simulink model "CML_Dyanmic_Sensory_Weighting"  (R2015a)
settings: Solver=ode4  SolverMode=MultiTasking  StartTime=0.0  StopTime=inf  FixedStep=BKIN_STEP_TIME  RelTol=1e-3
StartFcn:
  |  warndlg('Dexterit-E models cannot run under simulation. Please compile your model and run it from within Dexterit-E.');set_param(bdroot,'SimulationCommand','stop')
model workspace (MAT data in the model file):
  col_x = 1
  col_y = 2
  RADIUS_VIS = 3
  COLOR_INIT = 4
  START_TARGET_COL = 1
  DELAY_POST_TRIAL_COL = 17
  BKIN_STEP_TIME = 0.00025
  COLOR_MOVE = 5
  START_WAIT_TIME_COL = 2
  STIM_DUR_COL = 13
  MAX_MOVE_TIME_COL = 14
  HOLD_TIME_COL = 15
  E_START_TRIAL = 2
  E_START_REACHED = 4
  E_MOVED_EARLY = 21
  E_GO_CUE = 9
  E_MOVE_TIMEOUT = 23
  E_HOLDING_STILL = 12
  E_END_TRIAL = 14
  CONTROL_PT3_COL = 10
  STROKE_WIDTH = 6
  K_HAND_VEL = 1
  E_MOVE_ON = 10
  CUE_TYPE_COL = 6
  HAND_VIS_COL = 5
  K_HOLDTIME = 2
  K_ROBOT_RAMP_TIME = 3
  E_ROBOT_RETURN_TO_START = 33
  E_ENABLED_CONTROLLER = 31
  K_TIME_TO_START = 4
  E_RETURN_TO_START = 35
  E_HOLD_POS = 37
  E_INCREMENTING_TSTEP1 = 6
  E_INCREMENTING_TSTEP2 = 7
  E_INCREMENTING_TSTEP3 = 8
  CONTROL_PT0_COL = 7
  BKIN_KINEMATIC_FRAME_SIZE = 400
  E_NO_EVENT = 0
  E_BUTTON_ON = 40
  CONTROL_PTV1_COL = 8
  CONTROL_PTV2_COL = 9
  CONTROL_PTP1_COL = 11
  CONTROL_PTP2_COL = 12
  REACH_TARGET_COL = 3
  VIS_TARGET_COL = 4
  RADIUS_LOGICAL = 7
  FEEDBACK_TIME_COL = 16
  K_HAND_TARGET = 5
  E_SHOW_FEEDBACK = 16
  K_MIDPOINTY = 6
  K_MIDPOINT_Y = 6
  K_ARC_FDBK_TARGET = 7
  TEXT1 = 8
  TEXT2 = 9
  TEXT3 = 10
  K_CUE_TARGET = 8
  CONTINUE = 4
  TEXT4 = 11
  E_PAUSE = 41
libraries: slrtlib x10, Video x9, General x3, KINARM_general x3, KINARM_loads x2, xpcnilib x1
(part 2 of 2)

== matlab function CML_Dyanmic_Sensory_Weighting/BezierCurve/Bezier_fnc ==
  data: startxy input; segCount input; posV output; posP output; VCODE input; VCODE_mod output; t input; target_rows input; Ptarget_rows input; control_points input; col_xy input
function [posV,posP,VCODE_mod] = fcn(startxy,segCount,VCODE,t,target_rows,Ptarget_rows,control_points,col_xy)
%#codegen

%VCODE_mod = [VCODE; VCODE];
VCODE_mod = VCODE;


%startxy is the absolute starting point for the segment

%Vtarget_rows and Ptarget_rows share the same first target so we
%just have to ask about the remaining ones

%find all the nonzero (valid) control points
target_rows = target_rows(target_rows>0);
Ptarget_rows = Ptarget_rows(Ptarget_rows>0);

offsetX = 0;
offsetY = 0;
if segCount > 0 %(all(abs(startxy) > 0.01))
    
    %this is the starting (x,y) position for this segment in cm, i.e., "(0,0)"
    %the difference between this and the absolute segment starting position
    %gives us the offset
    startX = control_points(target_rows(1),col_xy(1));
    startY = control_points(target_rows(1),col_xy(2));
    
    offsetX = startxy(1)-(startX/100);
    offsetY = startxy(2)-(startY/100);
end



%clip t just in case!
if t < 0
    t = 0;
elseif t > 1;
    t = 1;
end

%t_hat = [0:0.001:1];

%reshape t from purely linear to sigmoidal, to nicely shape the speed
%k = 20;
%t = 1/(1+exp(-k*(t-0.5)));

%t is shared for both V and P, to keep the movements in sync
%since the net primary direction distance is the same, the movements should
%unfold in parallel
t = t-sin(2*pi*t)/(2*pi);  %use the bell-shaped velocity profile from the trajectory controller


%we will fill in the Bezier curve code here

if (length(target_rows) == 3)
    
%     %reshape t from purely linear to some nicely shaped speed following the
%     %2/3 power law?
%     x = ((1-t_hat).^2)*control_points(target_rows(1),col_xy(1)) + 2*(t_hat.*(1-t_hat))*control_points(target_rows(2),col_xy(1)) + (t_hat.^2)*control_points(target_rows(3),col_xy(1));
%     y = ((1-t_hat).^2)*control_points(target_rows(1),col_xy(2)) + 2*(t_hat.*(1-t_hat))*control_points(target_rows(2),col_xy(2)) + (t_hat.^2)*control_points(target_rows(3),col_xy(2));
%     xdot = 2*(1-t_hat)*(control_points(target_rows(2),col_xy(1))-control_points(target_rows(1),col_xy(1))) + 2*t_hat*(control_points(target_rows(3),col_xy(1))-control_points(target_rows(2),col_xy(1)));
%     ydot = 2*(1-t_hat)*(control_points(target_rows(2),col_xy(2))-control_points(target_rows(1),col_xy(2))) + 2*t_hat*(control_points(target_rows(3),col_xy(2))-control_points(target_rows(2),col_xy(2)));
%     xdotdot = 2*(control_points(target_rows(3),col_xy(1)) - 2*control_points(target_rows(2),col_xy(1)) + control_points(target_rows(1),col_xy(1)))*ones(size(t_hat));
%     ydotdot = 2*(control_points(target_rows(3),col_xy(2)) - 2*control_points(target_rows(2),col_xy(2)) + control_points(target_rows(1),col_xy(2)))*ones(size(t_hat));
%     curv = abs(xdot.*ydotdot - ydot.*xdotdot)./((xdot.^2 + ydot.^2).^1.5); %curvature along the bezier curve
%     arcvel = curv.^(-2/3);
    
    
    posV = ((1-t)^2)*control_points(target_rows(1),col_xy) + 2*(t*(1-t))*control_points(target_rows(2),col_xy) + (t^2)*control_points(target_rows(3),col_xy);
elseif (length(target_rows) == 4)
    
%     %reshape t from purely linear to some nicely shaped speed following the
%     %2/3 power law?
%     x = ((1-t_hat).^3)*control_points(target_rows(1),col_xy(1)) + 3*(t_hat.*(1-t_hat).^2)*control_points(target_rows(2),col_xy(1)) + 3*((1-t_hat).*(t_hat.^2))*control_points(target_rows(3),col_xy(1)) + (t_hat.^3)*control_points(target_rows(4),col_xy(1));
%     y = ((1-t_hat).^3)*control_points(target_rows(1),col_xy(2)) + 3*(t_hat.*(1-t_hat).^2)*control_points(target_rows(2),col_xy(2)) + 3*((1-t_hat).*(t_hat.^2))*control_points(target_rows(3),col_xy(2)) + (t_hat.^3)*control_points(target_rows(4),col_xy(2));
%     xdot = 3*((1-t_hat).^2)*(control_points(target_rows(2),col_xy(1))-control_points(target_rows(1),col_xy(1))) + 6*((1-t_hat).*t_hat)*(control_points(target_rows(3),col_xy(1))-control_points(target_rows(2),col_xy(1))) + 3*(t_hat.^2)*(control_points(target_rows(4),col_xy(1))-control_points(target_rows(3),col_xy(1)));
%     ydot = 3*((1-t_hat).^2)*(control_points(target_rows(2),col_xy(2))-control_points(target_rows(1),col_xy(2))) + 6*((1-t_hat).*t_hat)*(control_points(target_rows(3),col_xy(2))-control_points(target_rows(2),col_xy(2))) + 3*(t_hat.^2)*(control_points(target_rows(4),col_xy(2))-control_points(target_rows(3),col_xy(2)));
%     xdotdot = 6*(1-t_hat)*(control_points(target_rows(3),col_xy(1))-2*control_points(target_rows(2),col_xy(1))+control_points(target_rows(1),col_xy(1))) + 6*(t_hat)*(control_points(target_rows(4),col_xy(1))-2*control_points(target_rows(3),col_xy(1))+control_points(target_rows(2),col_xy(1)));
%     ydotdot = 6*(1-t_hat)*(control_points(target_rows(3),col_xy(2))-2*control_points(target_rows(2),col_xy(2))+control_points(target_rows(1),col_xy(2))) + 6*(t_hat)*(control_points(target_rows(4),col_xy(2))-2*control_points(target_rows(3),col_xy(2))+control_points(target_rows(2),col_xy(2)));
%     curv = abs(xdot.*ydotdot - ydot.*xdotdot)./((xdot.^2 + ydot.^2).^1.5); %curvature along the bezier curve
%     arcvel = curv.^(-2/3);

    
    posV = ((1-t)^3)*control_points(target_rows(1),col_xy) + 3*(t*(1-t)^2)*control_points(target_rows(2),col_xy) + 3*((t^2)*(1-t))*control_points(target_rows(3),col_xy) + (t^3)*control_points(target_rows(4),col_xy);
elseif (length(target_rows) == 2)

    %t = t-sin(2*pi*t)/(2*pi);  %use the bell-shaped velocity profile from the trajectory controller
    posV = (1-t)*control_points(target_rows(1),col_xy) + (t)*control_points(target_rows(2),col_xy);
else %length == 1
    
    posV = control_points(target_rows(1),col_xy);
    
end


if (length(Ptarget_rows) == 3)
    
    posP = ((1-t)^2)*control_points(Ptarget_rows(1),col_xy) + 2*(t*(1-t))*control_points(Ptarget_rows(2),col_xy) + (t^2)*control_points(Ptarget_rows(3),col_xy);
    
elseif (length(Ptarget_rows) == 4)
    
    posP = ((1-t)^3)*control_points(Ptarget_rows(1),col_xy) + 3*(t*(1-t)^2)*control_points(Ptarget_rows(2),col_xy) + 3*((t^2)*(1-t))*control_points(Ptarget_rows(3),col_xy) + (t^3)*control_points(Ptarget_rows(4),col_xy);
    
elseif (length(Ptarget_rows) == 2)

    posP = (1-t)*control_points(Ptarget_rows(1),col_xy) + (t)*control_points(Ptarget_rows(2),col_xy);
    
else %length == 1
    
    posP = control_points(Ptarget_rows(1),col_xy);
    
end

posV = posV/100;
posV(1) = posV(1)+offsetX;
posV(2) = posV(2)+offsetY;

posP = posP/100;
posP(1) = posP(1)+offsetX;
posP(2) = posP(2)+offsetY;

VCODE_mod(1,3) = posV(1); %convert to meters
VCODE_mod(1,4) = posV(2); %convert to meters

%we will not add the posP position to the VCODE, we will use the hand
%feedback cursor instead

%VCODE_mod(2,3) = posP(1); %convert to meters
%VCODE_mod(2,4) = posP(2); %convert to meters

== matlab function CML_Dyanmic_Sensory_Weighting/Subsystem/MATLAB Function ==
  data: pos input; VCODE_MOD output; VCODE input
function VCODE_MOD = fcn(pos,VCODE)
%#codegen

VCODE_MOD = VCODE;

VCODE_MOD(3) = pos(1);
VCODE_MOD(4) = pos(2);

== matlab function CML_Dyanmic_Sensory_Weighting/ShowHandPath/MATLAB Function ==
  data: Path input; npoints input; state input; VCODE output; VCODES input; startpos input; reachpos input; reachmidpoint_log output
function [VCODE,reachmidpoint_log]  = interp(Path,npoints,state, VCODES,startpos,reachpos)
%#codegen
VCODE = VCODES;
MAX_PATH_LENGTH = 25; % MUST BE ODD, maximum number of vertexes on a path

%{
interppts = zeros(1,MAX_PATH_LENGTH);

interval = npoints/(MAX_PATH_LENGTH);

interppts = [0:MAX_PATH_LENGTH-1]*interval+1;

interppts  = round(interppts);
if interppts(1) < 1
    interppts(1) = 1;
end
if interppts(end) >= npoints
    interppts(end) = npoints-1;
end
%}

% find desired points based on midpoint y values
% want to go backwards so its not pulling old values
MIDPOINT = (startpos(2)+reachpos(2))/2; % roughly
THRESH = 0.01; % larger for now
path_x = Path(1,:);
path_y = Path(2,:);
iMIDPOINT=-1; % as a catch
% brute force a for loop
%path_y_conditional = path_y>(MIDPOINT-THRESH) & path_y<(MIDPOINT+THRESH);
for ii =1:length(path_y)-1
    % use subtraction to look backwards
    testii = length(path_y)-ii;
    if path_y(testii)>(MIDPOINT-THRESH) && path_y(testii)<(MIDPOINT+THRESH)
        iMIDPOINT=testii;
        break
    end
end
% pull out y value closest to midpoint and use to get point
%iMIDPOINT = interp1(path_y,1:length(path_y),MIDPOINT, 'nearest');
% load interpath with nearest neighbors to iMIDPOINT
%interppts = zeros(25);
%interval = 1; % larger value = longer path, less refined
%interppts_start = iMIDPOINT-(round(MAX_PATH_LENGTH/2)-1)*interval;
%interppts = (interppts_start:interval:MAX_PATH_LENGTH);

%interppts=find(path_y>MIDPOINT-midthresh & path_y<MIDPOINT+midthresh); % set up conditional
% round it to have less points in the path
%interval=length(interppts)/(MAX_PATH_LENGTH);
%interppts = interppts(:,1:round(interval):end);

% apply mask
%interppath = Path(:,interppts);


%width=0.005;
width = 0.05;
colour = 65280;  %not sure how to set this?

% vcode      1 2 3 4 5 6      7     8 9   10 11 12 13 14 15 16
%path_code = [6 state 0 0 0 colour width 0 100 0  0  0  0  0  0  MAX_PATH_LENGTH];
% for one point circle
% vcode      1   2           3                  4           5      6     7
%path_code = [1 state path_x(iMIDPOINT) path_y(iMIDPOINT) colour colour width 0 100 width];
% test 
%path_code = [1 state 0.45 0.45 colour colour width 0 100 width];

%VCODE = zeros(1,70);
reachmidpoint_log = [path_x(iMIDPOINT), path_y(iMIDPOINT), iMIDPOINT];

if state > 0
    %VCODE(1,1:10) = path_code;
    VCODE(3:4) = [path_x(iMIDPOINT), path_y(iMIDPOINT)];
    %VCODE(1,17) = path_x(iMIDPOINT);
    %VCODE(1,18) = path_y(iMIDPOINT);
    %VCODE(1,17:2:66) = interppath(1,:);
    %VCODE(1,18:2:66) = interppath(2,:);
end

== matlab function CML_Dyanmic_Sensory_Weighting/Play Sound/Play sound over and over ==
  data: tone input; output output; beep input; beep1 input; beep2 input
function output = fcn(tone,beep,beep1,beep2)
%#codegen

persistent t last_tone_state
if isempty(t), t = 0; end
if isempty(last_tone_state), last_tone_state = 0; end

trigger = last_tone_state ~= tone;
if trigger > 0
    last_tone_state = tone;
end

output = 0;		% default
if t == 0 && trigger > 0
	% start the playing of the sound.
	t = t + 1;
end

if tone == 1
    data = beep;
elseif tone == 2
    data = beep1;
elseif tone == 3
    data = beep2;
else 
    t = 0;
    data = 0;
end

if t > 0
	output = data(t);
	if t == length(data)
		t = 0;
	else
		t = t + 1;
	end
end

== matlab function CML_Dyanmic_Sensory_Weighting/ShowHandPath/Bezier_fnc ==
  data: state input; startxy input; target_rows input; Ptarget_rows input; CueType input; VCODE output; control_points input; col_xy input
function VCODE  = fcn(state,startxy,target_rows,Ptarget_rows,CueType,control_points,col_xy)
%#codegen

t = [0:(1/24):1];

segCount = 1;

%startxy is the absolute starting point for the segment

%find all the nonzero (valid) control points
target_rows = target_rows(target_rows>0);
Ptarget_rows = Ptarget_rows(Ptarget_rows>0);

offsetX = 0;
offsetY = 0;
if segCount > 0 %(all(abs(startxy) > 0.01))
    
    %this is the starting (x,y) position for this segment in cm, i.e., "(0,0)"
    %the difference between this and the absolute segment starting position
    %gives us the offset
    startX = control_points(target_rows(1),col_xy(1));
    startY = control_points(target_rows(1),col_xy(2));
    
    offsetX = startxy(1)-(startX/100);
    offsetY = startxy(2)-(startY/100);
end


%we will fill in the Bezier curve code here

if (length(target_rows) == 3)
    
    posVx = ((1-t).^2)*control_points(target_rows(1),col_xy(1)) + 2*(t.*(1-t))*control_points(target_rows(2),col_xy(1)) + (t.^2)*control_points(target_rows(3),col_xy(1));
    posVy = ((1-t).^2)*control_points(target_rows(1),col_xy(2)) + 2*(t.*(1-t))*control_points(target_rows(2),col_xy(2)) + (t.^2)*control_points(target_rows(3),col_xy(2));
elseif (length(target_rows) == 4)
    
    posVx = ((1-t).^3)*control_points(target_rows(1),col_xy(1)) + 3*(t.*(1-t).^2)*control_points(target_rows(2),col_xy(1)) + 3*((t.^2).*(1-t))*control_points(target_rows(3),col_xy(1)) + (t.^3)*control_points(target_rows(4),col_xy(1));
    posVy = ((1-t).^3)*control_points(target_rows(1),col_xy(2)) + 3*(t.*(1-t).^2)*control_points(target_rows(2),col_xy(2)) + 3*((t.^2).*(1-t))*control_points(target_rows(3),col_xy(2)) + (t.^3)*control_points(target_rows(4),col_xy(2));
elseif (length(target_rows) == 2)

    posVx = (1-t)*control_points(target_rows(1),col_xy(1)) + (t)*control_points(target_rows(2),col_xy(1));
    posVy = (1-t)*control_points(target_rows(1),col_xy(2)) + (t)*control_points(target_rows(2),col_xy(2));
else %length == 1
    
    posVx = control_points(target_rows(1),col_xy(1));
    posVy = control_points(target_rows(1),col_xy(2));
    
end


if (length(Ptarget_rows) == 3)
    
    posPx = ((1-t).^2)*control_points(Ptarget_rows(1),col_xy(1)) + 2*(t.*(1-t))*control_points(Ptarget_rows(2),col_xy(1)) + (t.^2)*control_points(Ptarget_rows(3),col_xy(1));
    posPy = ((1-t).^2)*control_points(Ptarget_rows(1),col_xy(2)) + 2*(t.*(1-t))*control_points(Ptarget_rows(2),col_xy(2)) + (t.^2)*control_points(Ptarget_rows(3),col_xy(2));
    
elseif (length(Ptarget_rows) == 4)
    
    posPx = ((1-t).^3)*control_points(Ptarget_rows(1),col_xy(1)) + 3*(t.*(1-t).^2)*control_points(Ptarget_rows(2),col_xy(1)) + 3*((t.^2).*(1-t))*control_points(Ptarget_rows(3),col_xy(1)) + (t.^3)*control_points(Ptarget_rows(4),col_xy(1));
    posPy = ((1-t).^3)*control_points(Ptarget_rows(1),col_xy(2)) + 3*(t.*(1-t).^2)*control_points(Ptarget_rows(2),col_xy(2)) + 3*((t.^2).*(1-t))*control_points(Ptarget_rows(3),col_xy(2)) + (t.^3)*control_points(Ptarget_rows(4),col_xy(2));
elseif (length(Ptarget_rows) == 2)

    posPx = (1-t)*control_points(Ptarget_rows(1),col_xy(1)) + (t)*control_points(Ptarget_rows(2),col_xy(1));
    posPy = (1-t)*control_points(Ptarget_rows(1),col_xy(2)) + (t)*control_points(Ptarget_rows(2),col_xy(2));
else %length == 1
    
    posPx = control_points(Ptarget_rows(1),col_xy(1));
    posPy = control_points(Ptarget_rows(1),col_xy(2));
    
end

posVx = posVx/100;
posVy = posVy/100;
posVx = posVx+offsetX;
posVy = posVy+offsetY;

posPx = posPx/100;
posPy = posPy/100;
posPx = posPx+offsetX;
posPy = posPy+offsetY;


width = 0.005;
colour = 65280;  %not sure how to set this?

% vcode      1 2 3 4 5 6      7     8 9   10 11 12 13 14 15 16
path_code = [6 state 0 0 0 colour width 0 100 0  0  0  0  0  0  25];

VCODE = zeros(2,70);

if state > 0
    if CueType == 0
        VCODE(1,1:16) = path_code;
        VCODE(1,17:2:66) = posVx;
        VCODE(1,18:2:66) = posVy;
    elseif CueType == 1
        VCODE(1,1:16) = path_code;
        VCODE(1,17:2:66) = posPx;
        VCODE(1,18:2:66) = posPy;
    elseif CueType == 2
        VCODE(1,1:16) = path_code;
        VCODE(1,17:2:66) = posVx;
        VCODE(1,18:2:66) = posVy;

        VCODE(2,1:16) = path_code;
        VCODE(2,17:2:66) = posPx;
        VCODE(2,18:2:66) = posPy;
    end        
        
end



%we will not add the posP position to the VCODE, we will use the hand
%feedback cursor instead

%VCODE_mod(2,3) = posP(1); %convert to meters
%VCODE_mod(2,4) = posP(2); %convert to meters

== matlab function CML_Dyanmic_Sensory_Weighting/BezierFDBK/Bezier_fnc ==
  data: state input; startxy input; target_rows input; VCODE output; control_points input; col_xy input
function VCODE  = fcn(state,startxy,target_rows,control_points,col_xy)
%#codegen

t = [0:(1/24):1];

segCount = 1;
CueType=0;

%startxy is the absolute starting point for the segment

%find all the nonzero (valid) control points
target_rows = target_rows(target_rows>0);

offsetX = 0;
offsetY = 0;
if segCount > 0 %(all(abs(startxy) > 0.01))
    
    %this is the starting (x,y) position for this segment in cm, i.e., "(0,0)"
    %the difference between this and the absolute segment starting position
    %gives us the offset
    startX = control_points(target_rows(1),col_xy(1));
    startY = control_points(target_rows(1),col_xy(2));
    
    offsetX = startxy(1)-(startX/100);
    offsetY = startxy(2)-(startY/100);
end


%we will fill in the Bezier curve code here

if (length(target_rows) == 3)
    
    posVx = ((1-t).^2)*control_points(target_rows(1),col_xy(1)) + 2*(t.*(1-t))*control_points(target_rows(2),col_xy(1)) + (t.^2)*control_points(target_rows(3),col_xy(1));
    posVy = ((1-t).^2)*control_points(target_rows(1),col_xy(2)) + 2*(t.*(1-t))*control_points(target_rows(2),col_xy(2)) + (t.^2)*control_points(target_rows(3),col_xy(2));
elseif (length(target_rows) == 4)
    
    posVx = ((1-t).^3)*control_points(target_rows(1),col_xy(1)) + 3*(t.*(1-t).^2)*control_points(target_rows(2),col_xy(1)) + 3*((t.^2).*(1-t))*control_points(target_rows(3),col_xy(1)) + (t.^3)*control_points(target_rows(4),col_xy(1));
    posVy = ((1-t).^3)*control_points(target_rows(1),col_xy(2)) + 3*(t.*(1-t).^2)*control_points(target_rows(2),col_xy(2)) + 3*((t.^2).*(1-t))*control_points(target_rows(3),col_xy(2)) + (t.^3)*control_points(target_rows(4),col_xy(2));
elseif (length(target_rows) == 2)

    posVx = (1-t)*control_points(target_rows(1),col_xy(1)) + (t)*control_points(target_rows(2),col_xy(1));
    posVy = (1-t)*control_points(target_rows(1),col_xy(2)) + (t)*control_points(target_rows(2),col_xy(2));
else %length == 1
    
    posVx = control_points(target_rows(1),col_xy(1));
    posVy = control_points(target_rows(1),col_xy(2));
    
end


posVx = posVx/100;
posVy = posVy/100;
posVx = posVx+offsetX;
posVy = posVy+offsetY;

width = 0.005;
colour = 65280;  %not sure how to set this?

% vcode      1 2 3 4 5 6      7     8 9   10 11 12 13 14 15 16
path_code = [6 state 0 0 0 colour width 0 100 0  0  0  0  0  0  25];

VCODE = zeros(2,70);

if state > 0
    if CueType == 0
        VCODE(1,1:16) = path_code;
        VCODE(1,17:2:66) = posVx;
        VCODE(1,18:2:66) = posVy;
       %{
    elseif CueType == 1
        VCODE(1,1:16) = path_code;
        VCODE(1,17:2:66) = posPx;
        VCODE(1,18:2:66) = posPy;
    elseif CueType == 2
        VCODE(1,1:16) = path_code;
        VCODE(1,17:2:66) = posVx;
        VCODE(1,18:2:66) = posVy;

        VCODE(2,1:16) = path_code;
        VCODE(2,17:2:66) = posPx;
        VCODE(2,18:2:66) = posPy;
        %}
    end        
        
end



%we will not add the posP position to the VCODE, we will use the hand
%feedback cursor instead

%VCODE_mod(2,3) = posP(1); %convert to meters
%VCODE_mod(2,4) = posP(2); %convert to meters
